simulink model "battery_model_2RC_2S1P"  (R2025a)
settings: Solver=ode15s  StartTime=0.0  StopTime=3600  RelTol=1e-2  AbsTol=1e-3  EnableMultiTasking=on
libraries: fl_lib x19, nesl_utility x17, ee_lib x4, batteryecm_lib x2
settings Model: LastModifiedBy=ishikawa
settings SolverCC: AutoScaleAbsTol=off  AlgebraicLoopSolver=TrustRegion  MaxZcPerStep=1.0
settings DataIOCC: LimitDataPoints=on  MaxDataPoints=10000
settings OptimizationCC: ReuseModelBlockBuffer=off  LifeSpan=inf
settings DebuggingCC: UnconnectedInputMsg=warning  UnconnectedOutputMsg=warning  UnconnectedLineMsg=warning  AllowSymbolicDim=off  SFUnexpectedBacktrackingDiag=warning  SFNoUnconditionalDefaultTransitionDiag=warning  SFExecutionAtInitializationDiag=none  ArithmeticOperatorsInVariantConditions=warning
settings ModelReferenceCC: EnableRefExpFcnMdlSchedulingChecks=on
settings SFSimCC: SimUseLocalCustomCode=off  CustomCodeUndefinedFunction=UseInterfaceOnly
settings RTWCC: RTWUseLocalCustomCode=off  GPUComputeCapability=3.5  DLArmComputeVersion=19.05
settings CodeAppCC: StateflowObjectComments=on
settings GRTTargetCC: TargetLangStandard=C89/C90 (ANSI)
settings ConfigComp: CovMetricSettings=dw  CovSaveCumulativeToWorkspaceVar=on  CovSaveSingleToWorkspaceVar=on  CovExternalEMLEnable=off  CovSFcnEnable=off
settings SimscapeCC: SimscapeLogType=all  SimscapeLogSimulationStatistics=on  SimscapeLogDataHistory=10000.0

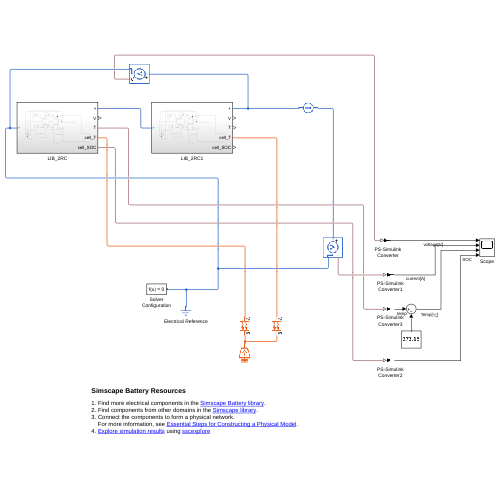
[thumbnail: Simulink's stored preview of the top-level diagram]
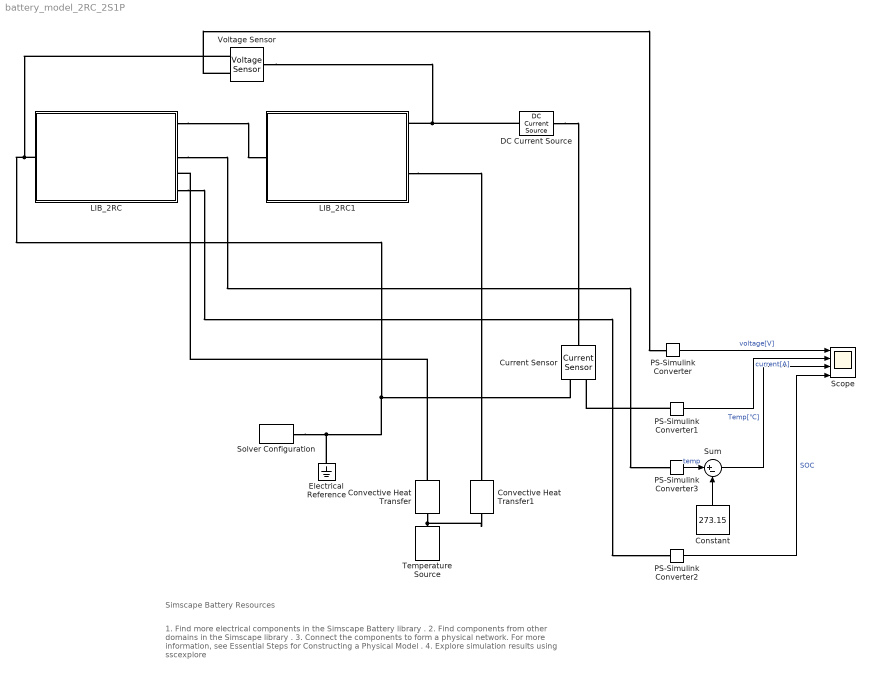
== system battery_model_2RC_2S1P ==
  note: 1. Find more electrical components in the Simscape Battery library .
      | 2. Find components from other domains in the Simscape library .
      | 3. Connect the components to form a physical network.
      | For more information, see Essential Steps for Constructing a Physical Model .
      | 4. Explore simulation results using sscexplore
  note: Simscape Battery Resources
  Constant : Constant  Value=273.15
  Convective Heat Transfer : fl_lib/Thermal/Thermal Elements/Convective Heat Transfer  thermal_type=foundation.enum.constant_variable.constant  area=4398.2 mm^2  heat_tr_coeff=20 W/(K*m^2)  min_heat_tr_coeff=1e-3 W/(K*m^2)  T_specify=off  T_priority=None  T=0 K  T_nominal_specify=off  T_nominal_value=1  T_nominal_unit=K  Q_specify=off  Q_priority=None  Q=0 W  Q_nominal_specify=off  Q_nominal_value=1  Q_nominal_unit=W
  Convective Heat Transfer1 : fl_lib/Thermal/Thermal Elements/Convective Heat Transfer  thermal_type=foundation.enum.constant_variable.constant  area=4398.2 mm^2  heat_tr_coeff=20 W/(K*m^2)  min_heat_tr_coeff=1e-3 W/(K*m^2)  T_specify=off  T_priority=None  T=0 K  T_nominal_specify=off  T_nominal_value=1  T_nominal_unit=K  Q_specify=off  Q_priority=None  Q=0 W  Q_nominal_specify=off  Q_nominal_value=1  Q_nominal_unit=W
  Current Sensor : fl_lib/Electrical/Electrical Sensors/Current Sensor
  DC Current Source : fl_lib/Electrical/Electrical Sources/DC Current Source  i0=5 A
      settings: InternalSimscapePortConfiguration="{\"Bottom\":[],\"Left\":[{\"id\":\"p\",\"label\":\"\",\"type\":\"foundation.electrical.electrical\"}],\"Right\":[{\"id\":\"n\",\"label\":\"\",\"type\":\"foundation.electrical.electrical\"}],\"Top\":[]}"
  Electrical Reference : fl_lib/Electrical/Electrical Elements/Electrical Reference
  LIB_2RC : Subsystem
  LIB_2RC1 : Subsystem
  PS-Simulink Converter{,1..3} (4 alike) : nesl_utility/PS-Simulink Converter  PhysicalDomain=network_engine_domain  SubClassName=ps_output  LeftPortType=input  RightPortType=output  PseudoPeriodic=off  Frequencies=[]  VectorFormat=inherit  Unit=inherit  AffineConversion=off
  Scope : Scope  NumInputPorts=4
      settings: ActiveDisplayYMinimum=3.6038991056085474  ActiveDisplayYMaximum=8.7134975618645871
  Solver Configuration : nesl_utility/Solver Configuration  PhysicalDomain=network_engine_domain  SubClassName=solver  LeftPortType=input  RightPortType=generic  Tones=[]  Harmonics=[]  SimulateNoise=off  Profile=off  UseLocalSampling=off  EnableSwitchedLinearOptims=on  FrequencyDomain=off  UseCCode=off  RelTol=0.001  AbsTol=1e-06  MinStep=1e-09  ToWorkspace=off  RevertToSquareIcSolve=off  NumHomotopyIterations=100  PhasorMode=off  PhasorModeNumHarmonics=1  ConsistencySolver=NEWTON_XTOL_AFTER_FTOL  IndexReductionMethod=DerivativeReplacement  DoDC=off  ResidualTolerance=1e-09  ConsistencyTolSource=GLOBAL  ConsistencyAbsTol=0.001  ConsistencyRelTol=0.001  ConsistencyTolFactor=0.001  UseLocalSolver=off  LocalSolverChoice=NE_BACKWARD_EULER_ADVANCER  ResolveIndetEquations=on  FunctionEvalNumThread=1  LocalSolverSampleTime=0.001  DoFixedCost=off  MaxNonlinIter=3  MaxModeIter=2  ComputeImpulses=off  ImpulseIterations=2  LinearAlgebra=auto  LinearAlgebraNumThread=0  EquationFormulation=NE_TIME_EF  DelaysMemoryBudget=1024  AutomaticFiltering=on  FilteringTimeConstant=0.001  PartitionStorageMethod=AS_NEEDED  PartitionMemoryBudget=1024  PartitionMethod=ROBUST  MultibodyUseLocalSolver=off  MultibodyLocalSolverChoice=ODE1  MultibodyLocalSolverSampleTime=0.001
  Sum : Sum  Inputs=|+-
  Temperature Source : fl_lib/Thermal/Thermal Sources/Temperature Source  temperature=298.15 K
  Voltage Sensor : fl_lib/Electrical/Electrical Sensors/Voltage Sensor
  wires:
  PS-Simulink Converter/1 -> Scope/1  "voltage[V]"
  PS-Simulink Converter1/1 -> Scope/2  "current[A]"
  PS-Simulink Converter2/1 -> Scope/4  "SOC"
  PS-Simulink Converter3/1 -> Sum/1  "temp"
  Constant/1 -> Sum/2
  Sum/1 -> Scope/3  "Temp[℃]"
  connections:
  Solver Configuration/RConn1 -- Electrical Reference/LConn1 -- Voltage Sensor/RConn2 -- LIB_2RC/LConn1 -- Current Sensor/RConn2
  PS-Simulink Converter1/LConn1 -- Current Sensor/RConn1
  DC Current Source/LConn1 -- Current Sensor/LConn1
  Convective Heat Transfer/RConn1 -- Convective Heat Transfer1/RConn1 -- Temperature Source/LConn1
  LIB_2RC/RConn3 -- PS-Simulink Converter3/LConn1
  Convective Heat Transfer/LConn1 -- LIB_2RC/RConn4
  LIB_2RC/RConn5 -- PS-Simulink Converter2/LConn1
  LIB_2RC/RConn1 -- LIB_2RC1/LConn1
  DC Current Source/RConn1 -- Voltage Sensor/LConn1 -- LIB_2RC1/RConn1
  Voltage Sensor/RConn1 -- PS-Simulink Converter/LConn1
  LIB_2RC1/RConn4 -- Convective Heat Transfer1/LConn1

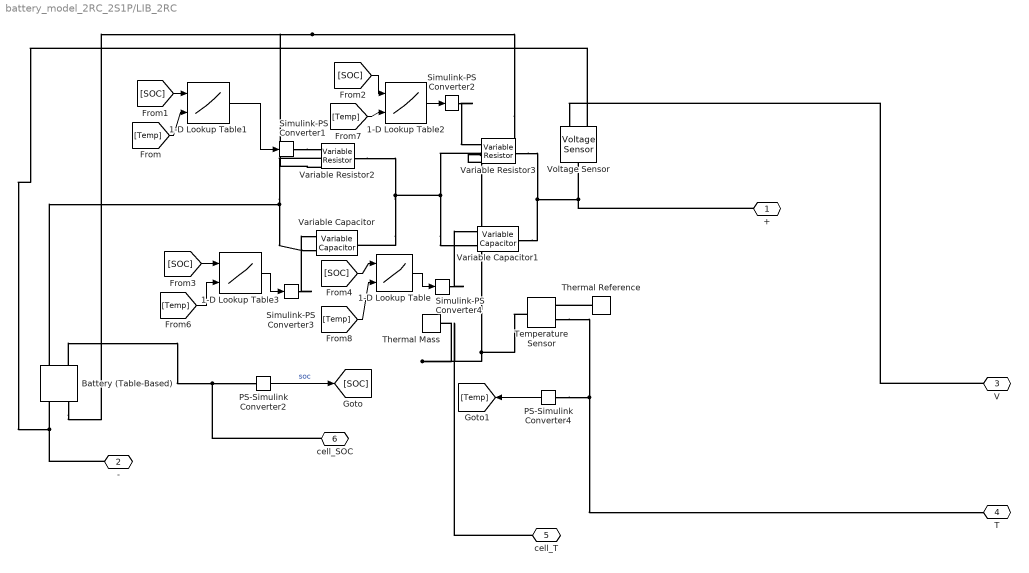
== system battery_model_2RC_2S1P/LIB_2RC ==
  1-D Lookup Table : Lookup_n-D  BreakpointsForDimension1=[0.2;0.3;0.4;0.5;0.6;0.7;0.8]  BreakpointsForDimension2=[243.15;253.15;263.15;273.15;293.15;313.15;333.15]  Table=[397.027539766071 413.310716720776 450.288774751873 484.819114610467 708.496704080481 1018.18115313393 1458.65326678376;424.160278757141 453.825413446659 523.404522348996 631.9600040269009 947.03250742128 1493.43845540211 2217.48074264787;445.080170656404 486.033224095827 563.317756801399 683.004425228606 1038.61139579099 1674.11304631932 2558.22434329923;455.398203100465 496.827822276761 571.533663638549 690.280792821343 1055.52640859521 1694.30417810877 2606.65823475404;450.805024482046 491.645093905588 567.6042393287059 687.869379202455 958.88347532501 1503.12492310199 2245.84613474158;459.20425063845 505.517182572026 566.7462150739819 674.399780009527 1012.81365894071 1541.62099228793 2186.17014175407;440.690556106675 465.368272327513 510.221909646828 603.247409685859 936.9228291323921 1585.76440619997 2335.62274337301]  InterpMethod=Cubic spline  ExtrapMethod=Cubic spline  InternalRulePriority=Speed  RndMeth=Simplest
      settings: InputPortMap=u0,u1
  1-D Lookup Table1 : Lookup_n-D  BreakpointsForDimension1=[0.1;0.2;0.3;0.4;0.5;0.6;0.7;0.8;0.9]  BreakpointsForDimension2=[243.15;253.15;263.15;273.15;293.15;313.15;333.15]  Table=[0.0648840256616996 0.0548544229488452 0.0410756789651543 0.00365935665197351 0.00410447217653615 0.0042287075329693 0.00446198100466879;0.000100000000000031 0.000185860329266272 0.00063291627023489 0.000604389587689878 0.00159168669392803 0.0016313368228375 0.00200106459466915;0.000100000000000657 0.000178858598639097 0.000694707150185237 0.00125188824704277 0.00176891372610466 0.00209070161735659 0.00247958451818985;0.000100000000001458 0.000100000085659489 0.000423782841219483 0.000938984921591674 0.00141231326940913 0.00167345242239196 0.00202829350359598;0.000100000000005779 0.000100000434574669 0.000364143335480069 0.0009126326610232501 0.00147302896089186 0.00170156587463233 0.0020630219200505;0.000100000000000059 0.000278496083040111 0.000932087348991903 0.00158899396065768 0.00191094085461356 0.00241949669919031 0.00294718757231742;0.000157820659890285 0.00106750348889988 0.00170837536179057 0.00230532371700022 0.00287920920827158 0.00321022629451256 0.00313048840253092;0.00177370275978769 0.00220599934990951 0.00213979379110787 0.00196046296256981 0.00192605061749151 0.00211861368543494 0.00233113190320715;0.000100000002763379 0.000100000000000054 0.000100000000653121 0.0001 0.008148072217938821 0.000704666332425065 0.00115546872752894]  InternalRulePriority=Speed  RndMeth=Simplest
      settings: InputPortMap=u0,u1
  1-D Lookup Table2 : Lookup_n-D  BreakpointsForDimension1=[0.1;0.2;0.3;0.4;0.5;0.6;0.7;0.8;0.9]  BreakpointsForDimension2=[243.15;253.15;263.15;273.15;293.15;313.15;333.15]  Table=[0.0312362200904875 0.0315941026250706 0.0325412525306707 0.06566459208756791 0.0513687856330062 0.0398557955825684 0.0352414860805867;0.0583154306341024 0.0541889718032672 0.0485485115411798 0.0405853877005846 0.0253230417200522 0.0179009478462281 0.014307904930947;0.0536064189215573 0.0500390783463631 0.0433999709749259 0.0362267299181839 0.0236360991500641 0.0163691636487888 0.0130777917670481;0.0510050016137325 0.0473244390449334 0.0406214407925902 0.0337999790008502 0.0217500314411443 0.014239465970092 0.0108482476470579;0.0489305258721882 0.0456158921911874 0.0395186949619077 0.032565240420024 0.0203018907734851 0.0132138263566234 0.0100754346546588;0.052109451999107 0.049581529928274 0.0435904805430911 0.0359457745514755 0.0223175296306251 0.0168395096404479 0.0145466336811264;0.0464891543332739 0.0461866422714133 0.0413831033248225 0.0343229536328831 0.0214923117112032 0.0152124572665625 0.012597749276845;0.0507650491686061 0.0490964567145729 0.0447555398141767 0.0371516971280947 0.0236401140020694 0.0168783192334412 0.0134119198713262;0.0485073831147304 0.0352842403123327 0.0287671376669305 0.0265741690411721 0.0113474189770295 0.0120077119241438 0.00910795807643172]  InternalRulePriority=Speed  RndMeth=Simplest
      settings: InputPortMap=u0,u1
  1-D Lookup Table3 : Lookup_n-D  BreakpointsForDimension1=[0.1;0.2;0.3;0.4;0.5;0.6;0.7;0.8;0.9]  BreakpointsForDimension2=[243.15;253.15;263.15;273.15;293.15;313.15;333.15]  Table=[424.737364805381 483.271376452374 636.374167822421 110.165370185585 210.959116483621 313.2910014267 429.704220236589;52.6100971695542 105.248860126284 63.6650097826792 60.5918177276404 590.998027541052 996.160700447975 1154.49089964508;90.42580825145249 312.74974100652 48.6954548231183 44.3380567111186 357.175111931739 582.326548341105 771.438129167261;118.248383199082 99.28484606029799 166.076514539697 33.3725870856565 424.226062352995 719.387999873913 951.14636655943;918.679938144521 17.7650082120618 162.910459604258 69.3161002074154 489.546217553075 740.276114872735 939.308771982209;2.33207460618265 21.5530951458301 3.6964219785336 146.524187256498 348.153708802123 510.139939288567 656.967471434281;531.457927571111 27.4074025424315 2.72381788457468 199.034282888046 301.850047314288 496.97606871071 792.228617026462;17.756055458357 149.39468287018 289.425440553852 448.824396398649 673.5667264432579 937.09993120302 1096.43767182893;134.492899453975 350.115225919153 316.422261704154 264.245690439253 3346.03757120953 1441.63234506984 1579.79386522281]  InternalRulePriority=Speed  RndMeth=Simplest
      settings: InputPortMap=u0,u1
  Battery (Table-Based) : batteryecm_lib/Battery (Table-Based)  SOC_vec=[0, .2, .4, .6, .8, 1 ]  T_dependence=simscape.enum.tablebattery.temperature_dependence.yes  prm_dir=simscape.enum.tablebattery.prm_dir.noCurrentDirectionality  T_vec=[243.15, 273.15, 333.15] K  V0_mat="[2.5, 2.5, 2.5; 3.42101188834904, 3.429363958294, 3.43097550824307; 3.59742438009383, 3.61108748742895, 3.6176423842731; 3.78966665741075, 3.80246978402262, 3.81751594086923;  4.00549793710987, 4.02037931005492, 4.02637725260671; 4.2, 4.2, 4.2] V"  V0_vec=[3.5057, 3.566, 3.6337, 3.7127, 3.9259, 4.0777, 4.1928] V  V_range=[0, inf] V  R0_mat=[0.14, 0.053, 0.008; 0.129999964197049, 0.0446688648295249, 0.00668298362381311; 0.116587668750708, 0.0373578823461791, 0.00550858692009345; 0.108099281225994, 0.0323106583204613, 0.00506405532754667; 0.104972042746652, 0.0314197816681482, 0.00495762078874784; 0.105, 0.031, 0.00495 ] Ohm  R0_vec=[.0085, .0085, .0087, .0082, .0083, .0085, .0085] Ohm  R0_dis_mat=[.0117, .0085, .009; .011, .0085, .009; .0114, .0087, .0092; .0107, .0082, .0088; .0107, .0083, .0091; .0113, .0085, .0089; .0116, .0085, .0089] Ohm  R0_dis_vec=[.0085, .0085, .0087, .0082, .0083, .0085, .0085] Ohm  R0_ch_mat=[.0117, .0085, .009; .011, .0085, .009; .0114, .0087, .0092; .0107, .0082, .0088; .0107, .0083, .0091; .0113, .0085, .0089; .0116, .0085, .0089] Ohm  R0_ch_vec=[.0085, .0085, .0087, .0082, .0083, .0085, .0085] Ohm  AH=5 A*hr  prm_leak=simscape.enum.tablebattery.prm_leak.disabled  Rleak_vec=[8000, 7000, 6000] Ohm  Rleak=7e3 Ohm  extrapolation_option=simscape.enum.extrapolation.nearest  SOC_port=simscape.enum.tablebattery.enable.yes  prm_dyn=simscape.enum.tablebattery.prm_dyn.off  R1_mat=[.0109, .0029, .0013; .0069, .0024, .0012; .0047, .0026, .0013; .0034, .0016, .001; .0033, .0023, .0014; .0033, .0018, .0011; .0028, .0017, .0011] Ohm  R1_vec=[.0029, .0024, .0026, .0016, .0023, .0018, .0017] Ohm  tau1_mat=[20, 36, 39; 31, 45, 39; 109, 105, 61; 36, 29, 26; 59, 77, 67; 40, 33, 29; 25, 39, 33] s  tau1_vec=[36, 45, 105, 29, 77, 33, 39] s  R2_mat=[.0109, .0029, .0013; .0069, .0024, .0012; .0047, .0026, .0013; .0034, .0016, .001; .0033, .0023, .0014; .0033, .0018, .0011; .0028, .0017, .0011] Ohm  R2_vec=[.0029, .0024, .0026, .0016, .0023, .0018, .0017] Ohm  tau2_mat=[20, 36, 39; 31, 45, 39; 109, 105, 61; 36, 29, 26; 59, 77, 67; 40, 33, 29; 25, 39, 33] s  tau2_vec=[36, 45, 105, 29, 77, 33, 39] s  R3_mat=[.0109, .0029, .0013; .0069, .0024, .0012; .0047, .0026, .0013; .0034, .0016, .001; .0033, .0023, .0014; .0033, .0018, .0011; .0028, .0017, .0011] Ohm  R3_vec=[.0029, .0024, .0026, .0016, .0023, .0018, .0017] Ohm  tau3_mat=[20, 36, 39; 31, 45, 39; 109, 105, 61; 36, 29, 26; 59, 77, 67; 40, 33, 29; 25, 39, 33] s  tau3_vec=[36, 45, 105, 29, 77, 33, 39] s  R4_mat=[.0109, .0029, .0013; .0069, .0024, .0012; .0047, .0026, .0013; .0034, .0016, .001; .0033, .0023, .0014; .0033, .0018, .0011; .0028, .0017, .0011] Ohm  R4_vec=[.0029, .0024, .0026, .0016, .0023, .0018, .0017] Ohm  tau4_mat=[20, 36, 39; 31, 45, 39; 109, 105, 61; 36, 29, 26; 59, 77, 67; 40, 33, 29; 25, 39, 33] s  tau4_vec=[36, 45, 105, 29, 77, 33, 39] s  R5_mat=[.0109, .0029, .0013; .0069, .0024, .0012; .0047, .0026, .0013; .0034, .0016, .001; .0033, .0023, .0014; .0033, .0018, .0011; .0028, .0017, .0011] Ohm  R5_vec=[.0029, .0024, .0026, .0016, .0023, .0018, .0017] Ohm  tau5_mat=[20, 36, 39; 31, 45, 39; 109, 105, 61; 36, 29, 26; 59, 77, 67; 40, 33, 29; 25, 39, 33] s  tau5_vec=[36, 45, 105, 29, 77, 33, 39] s  prm_fade=simscape.enum.tablebattery.prm_fade.equations  N0=100  dV0=0  dR0=0  dAH=0  dRleak=0  dR1=0  dR2=0  dR3=0  dR4=0  dR5=0  N0vec=[100, 200, 300]  Tfadevec=[298.15, 323.15] K  dV0vec=[0, 0, 0]  dR0vec=[0, 0, 0]  dAHvec=[0, 0, 0]  dRleakvec=[0, 0, 0]  dR1vec=[0, 0, 0]  dR2vec=[0, 0, 0]  dR3vec=[0, 0, 0]  dR4vec=[0, 0, 0]  dR5vec=[0, 0, 0]  dV0mat=[0, 0; 0, 0; 0, 0]  dR0mat=[0, 0; 0, 0; 0, 0]  dAHmat=[0, 0; 0, 0; 0, 0]  dRleakmat=[0, 0; 0, 0; 0, 0]  dR1mat=[0, 0; 0, 0; 0, 0]  dR2mat=[0, 0; 0, 0; 0, 0]  dR3mat=[0, 0; 0, 0; 0, 0]  dR4mat=[0, 0; 0, 0; 0, 0]  dR5mat=[0, 0; 0, 0; 0, 0]  prm_age_modeling=simscape.enum.tablebattery.prm_age_modeling.equation  storage_dt_age_vec=[0] d  storage_T_age_vec=[273] K  prm_age_OCV=simscape.enum.tablebattery.prm_age_OCV.OCV  OCV_age=0.9  SOC_age=0.6  prm_age_resistance=simscape.enum.tablebattery.prm_age.disabled  OCV_scaling_age_resistance=2.2134e6  OCV_offset_age_resistance=1.632e6  temp_exp_age_resistance=0.515833569 V  t_exp_age_resistance=0.75  T_age_vec_resistance=[273.15, 298.15, 323.15] K  dt_age_vec_resistance=[90, 180, 270, 360] d  dR0_age_vec=[0, 0, 0]  t_meas_dR0_age=100 d  dR0_age_mat=[0, 0, 0; 0, 0, 0; 0, 0, 0; 0, 0, 0]  prm_age_capacity=simscape.enum.tablebattery.prm_age.disabled  OCV_scaling_age_capacity=1.5097e07  OCV_offset_age_capacity=8.3625e06  temp_exp_age_capacity=0.6011 V  t_exp_age_capacity=0.75  T_age_vec_capacity=[273.15, 298.15, 323.15] K  dt_age_vec_capacity=[90, 180, 270, 360] d  dAH_age_vec=[0, 0, 0]  t_meas_dAH_age=100 d  dAH_age_mat=[0, 0, 0; 0, 0, 0; 0, 0, 0; 0, 0, 0]  thermal_port=simscape.enum.thermaleffects.model  temperature=298.15 K  thermal_mass=1 J/K  i_specify=off  i_priority=None  i=0 A  i_nominal_specify=off  i_nominal_value=1  i_nominal_unit=A  v_specify=off  v_priority=None  v=0 V  v_nominal_specify=off  v_nominal_value=1  v_nominal_unit=V  stateOfCharge_specify=on  stateOfCharge_priority=High  stateOfCharge=1  stateOfCharge_nominal_specify=on  stateOfCharge_nominal_value=1  stateOfCharge_nominal_unit=1  num_cycles_specify=off  num_cycles_priority=High  num_cycles=0  num_cycles_nominal_specify=off  num_cycles_nominal_value=1  num_cycles_nominal_unit=1  cell_temperature_specify=on  cell_temperature_priority=High  cell_temperature=298.15 K  cell_temperature_nominal_specify=off  cell_temperature_nominal_value=1  cell_temperature_nominal_unit=K
  PS-Simulink Converter2 : nesl_utility/PS-Simulink Converter  PhysicalDomain=network_engine_domain  SubClassName=ps_output  LeftPortType=input  RightPortType=output  PseudoPeriodic=off  Frequencies=[]  VectorFormat=inherit  Unit=inherit  AffineConversion=off
  PS-Simulink Converter4 : nesl_utility/PS-Simulink Converter  PhysicalDomain=network_engine_domain  SubClassName=ps_output  LeftPortType=input  RightPortType=output  PseudoPeriodic=off  Frequencies=[]  VectorFormat=inherit  Unit=inherit  AffineConversion=off
  Simulink-PS Converter{1..4} (4 alike) : nesl_utility/Simulink-PS Converter  PhysicalDomain=network_engine_domain  SubClassName=ps_input  LeftPortType=input  RightPortType=output  PseudoPeriodic=off  Frequencies=[]  NoiseDistribution=none  NoiseParameters=[]  Unit=1  AffineConversion=off  FilteringAndDerivatives=provide  SimscapeFilterOrder=1  InputFilterTimeConstant=0.001  UdotUserProvided=0
  Temperature Sensor : fl_lib/Thermal/Thermal Sensors/Temperature Sensor  temperature_measure=foundation.enum.MeasurementReference.difference
  Thermal Mass : fl_lib/Thermal/Thermal Elements/Thermal Mass  mass_type=foundation.enum.constant_variable.constant  mass=67.9 g  sp_heat=900 J/(K*kg)  mass_min=1e-6 kg  num_ports=foundation.enum.numPorts2.one  m_specify=off  m_priority=High  m=1 kg  m_nominal_specify=off  m_nominal_value=1  m_nominal_unit=kg  T_specify=off  T_priority=High  T=300 K  T_nominal_specify=off  T_nominal_value=1  T_nominal_unit=K  Q_specify=off  Q_priority=None  Q=0 W  Q_nominal_specify=off  Q_nominal_value=1  Q_nominal_unit=W
  Thermal Reference : fl_lib/Thermal/Thermal Elements/Thermal Reference
  Variable Capacitor : ee_lib/Passive/Variable Capacitor  prm=2  Cmin=1e-9 F  r=1e-6 Ohm  v0=0 V  q0=0 C
      settings: InternalSimscapePortConfiguration="{\"Bottom\":[],\"Left\":[{\"id\":\"C\",\"label\":\"C\",\"type\":\"input\"},{\"id\":\"p\",\"label\":\"+\",\"type\":\"foundation.electrical.electrical\"}],\"Right\":[{\"id\":\"n\",\"label\":\"-\",\"type\":\"foundation.electrical.electrical\"}],\"Top\":[]}"
  Variable Capacitor1 : ee_lib/Passive/Variable Capacitor  prm=2  Cmin=1e-9 F  r=1e-6 Ohm  v0=0 V  q0=0 C
      settings: InternalSimscapePortConfiguration="{\"Bottom\":[],\"Left\":[{\"id\":\"C\",\"label\":\"C\",\"type\":\"input\"},{\"id\":\"p\",\"label\":\"+\",\"type\":\"foundation.electrical.electrical\"}],\"Right\":[{\"id\":\"n\",\"label\":\"-\",\"type\":\"foundation.electrical.electrical\"}],\"Top\":[]}"
  Variable Resistor2 : fl_lib/Electrical/Electrical Elements/Variable Resistor  Rmin=0 Ohm  thermalEnable=true  thermal_mass=1 J/K  i_specify=off  i_priority=None  i=0 A  i_nominal_specify=off  i_nominal_value=1  i_nominal_unit=A  v_specify=off  v_priority=None  v=0 V  v_nominal_specify=off  v_nominal_value=1  v_nominal_unit=V  T_specify=off  T_priority=None  T=300 K  T_nominal_specify=off  T_nominal_value=1  T_nominal_unit=K
      settings: InternalSimscapePortConfiguration="{\"Bottom\":[],\"Left\":[{\"id\":\"R\",\"label\":\"R\",\"type\":\"input\"},{\"id\":\"p\",\"label\":\"+\",\"type\":\"foundation.electrical.electrical\"}],\"Right\":[{\"id\":\"n\",\"label\":\"-\",\"type\":\"foundation.electrical.electrical\"}],\"Top\":[{\"id\":\"H\",\"label\":\"H\",\"type\":\"foundation.thermal.thermal\"}]}"
  Variable Resistor3 : fl_lib/Electrical/Electrical Elements/Variable Resistor  Rmin=0 Ohm  thermalEnable=true  thermal_mass=1 J/K  i_specify=off  i_priority=None  i=0 A  i_nominal_specify=off  i_nominal_value=1  i_nominal_unit=A  v_specify=off  v_priority=None  v=0 V  v_nominal_specify=off  v_nominal_value=1  v_nominal_unit=V  T_specify=off  T_priority=None  T=300 K  T_nominal_specify=off  T_nominal_value=1  T_nominal_unit=K
      settings: InternalSimscapePortConfiguration="{\"Bottom\":[],\"Left\":[{\"id\":\"R\",\"label\":\"R\",\"type\":\"input\"},{\"id\":\"p\",\"label\":\"+\",\"type\":\"foundation.electrical.electrical\"}],\"Right\":[{\"id\":\"n\",\"label\":\"-\",\"type\":\"foundation.electrical.electrical\"}],\"Top\":[{\"id\":\"H\",\"label\":\"H\",\"type\":\"foundation.thermal.thermal\"}]}"
  Voltage Sensor : fl_lib/Electrical/Electrical Sensors/Voltage Sensor
  + : PMIOPort  Side=Right
  - : PMIOPort  Port=2  Side=Left
  V : PMIOPort  Port=3  Side=Right
  T : PMIOPort  Port=4  Side=Right
  cell_T : PMIOPort  Port=5  Side=Right
  cell_SOC : PMIOPort  Port=6  Side=Right
  wires:
  [SOC] -> 1-D Lookup Table/1
  1-D Lookup Table1/1 -> Simulink-PS Converter1/1
  PS-Simulink Converter4/1 -> [Temp]
  [Temp] -> 1-D Lookup Table3/2
  [SOC] -> 1-D Lookup Table2/1
  [SOC] -> 1-D Lookup Table1/1
  1-D Lookup Table3/1 -> Simulink-PS Converter3/1
  [SOC] -> 1-D Lookup Table3/1
  [Temp] -> 1-D Lookup Table1/2
  [Temp] -> 1-D Lookup Table2/2
  [Temp] -> 1-D Lookup Table/2
  PS-Simulink Converter2/1 -> [SOC]  "soc"
  1-D Lookup Table2/1 -> Simulink-PS Converter2/1
  1-D Lookup Table/1 -> Simulink-PS Converter4/1
  connections:
  Battery (Table-Based)/LConn2 -- cell_SOC/RConn1 -- PS-Simulink Converter2/LConn1
  Variable Capacitor/LConn2 -- Battery (Table-Based)/LConn1 -- Variable Resistor2/LConn2
  Temperature Sensor/RConn2 -- T/RConn1 -- PS-Simulink Converter4/LConn1
  -/RConn1 -- Voltage Sensor/RConn2 -- Battery (Table-Based)/RConn1
  V/RConn1 -- Voltage Sensor/RConn1
  Simulink-PS Converter3/RConn1 -- Variable Capacitor/LConn1
  Simulink-PS Converter4/RConn1 -- Variable Capacitor1/LConn1
  Thermal Reference/LConn1 -- Temperature Sensor/RConn1
  Variable Resistor3/LConn2 -- Variable Capacitor/RConn1 -- Variable Resistor2/RConn1 -- Variable Capacitor1/LConn2
  Simulink-PS Converter1/RConn1 -- Variable Resistor2/LConn1
  Simulink-PS Converter2/RConn1 -- Variable Resistor3/LConn1
  Variable Capacitor1/RConn1 -- Variable Resistor3/RConn1 -- +/RConn1 -- Voltage Sensor/LConn1
  Variable Resistor3/LConn3 -- Variable Resistor2/LConn3 -- Battery (Table-Based)/RConn2 -- Temperature Sensor/LConn1 -- cell_T/RConn1 -- Thermal Mass/LConn1

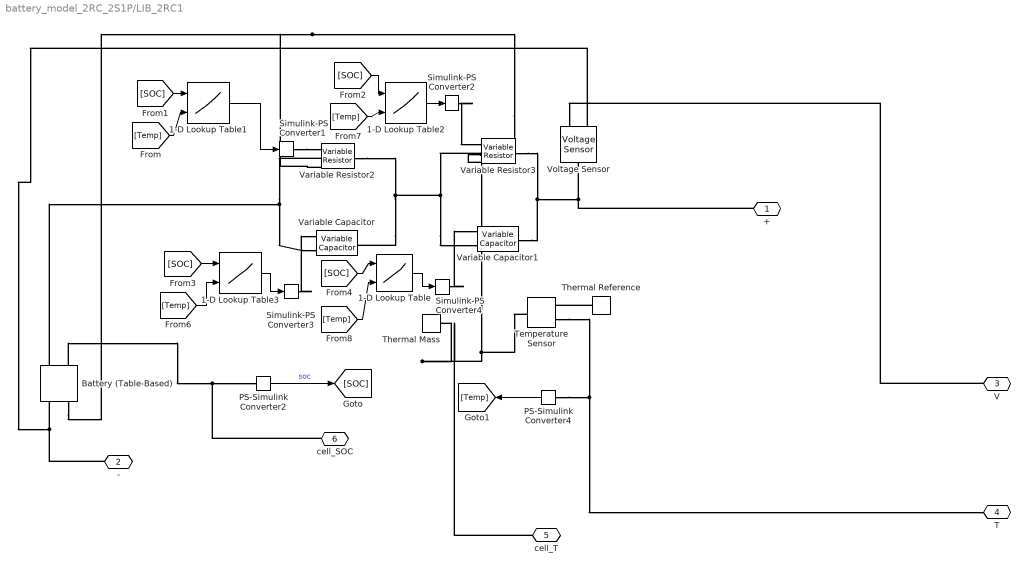
== system battery_model_2RC_2S1P/LIB_2RC1 ==
  1-D Lookup Table : Lookup_n-D  BreakpointsForDimension1=[0.2;0.3;0.4;0.5;0.6;0.7;0.8]  BreakpointsForDimension2=[243.15;253.15;263.15;273.15;293.15;313.15;333.15]  Table=[397.027539766071 413.310716720776 450.288774751873 484.819114610467 708.496704080481 1018.18115313393 1458.65326678376;424.160278757141 453.825413446659 523.404522348996 631.9600040269009 947.03250742128 1493.43845540211 2217.48074264787;445.080170656404 486.033224095827 563.317756801399 683.004425228606 1038.61139579099 1674.11304631932 2558.22434329923;455.398203100465 496.827822276761 571.533663638549 690.280792821343 1055.52640859521 1694.30417810877 2606.65823475404;450.805024482046 491.645093905588 567.6042393287059 687.869379202455 958.88347532501 1503.12492310199 2245.84613474158;459.20425063845 505.517182572026 566.7462150739819 674.399780009527 1012.81365894071 1541.62099228793 2186.17014175407;440.690556106675 465.368272327513 510.221909646828 603.247409685859 936.9228291323921 1585.76440619997 2335.62274337301]  InterpMethod=Cubic spline  ExtrapMethod=Cubic spline  InternalRulePriority=Speed  RndMeth=Simplest
      settings: InputPortMap=u0,u1
  1-D Lookup Table1 : Lookup_n-D  BreakpointsForDimension1=[0.1;0.2;0.3;0.4;0.5;0.6;0.7;0.8;0.9]  BreakpointsForDimension2=[243.15;253.15;263.15;273.15;293.15;313.15;333.15]  Table=[0.0648840256616996 0.0548544229488452 0.0410756789651543 0.00365935665197351 0.00410447217653615 0.0042287075329693 0.00446198100466879;0.000100000000000031 0.000185860329266272 0.00063291627023489 0.000604389587689878 0.00159168669392803 0.0016313368228375 0.00200106459466915;0.000100000000000657 0.000178858598639097 0.000694707150185237 0.00125188824704277 0.00176891372610466 0.00209070161735659 0.00247958451818985;0.000100000000001458 0.000100000085659489 0.000423782841219483 0.000938984921591674 0.00141231326940913 0.00167345242239196 0.00202829350359598;0.000100000000005779 0.000100000434574669 0.000364143335480069 0.0009126326610232501 0.00147302896089186 0.00170156587463233 0.0020630219200505;0.000100000000000059 0.000278496083040111 0.000932087348991903 0.00158899396065768 0.00191094085461356 0.00241949669919031 0.00294718757231742;0.000157820659890285 0.00106750348889988 0.00170837536179057 0.00230532371700022 0.00287920920827158 0.00321022629451256 0.00313048840253092;0.00177370275978769 0.00220599934990951 0.00213979379110787 0.00196046296256981 0.00192605061749151 0.00211861368543494 0.00233113190320715;0.000100000002763379 0.000100000000000054 0.000100000000653121 0.0001 0.008148072217938821 0.000704666332425065 0.00115546872752894]  InternalRulePriority=Speed  RndMeth=Simplest
      settings: InputPortMap=u0,u1
  1-D Lookup Table2 : Lookup_n-D  BreakpointsForDimension1=[0.1;0.2;0.3;0.4;0.5;0.6;0.7;0.8;0.9]  BreakpointsForDimension2=[243.15;253.15;263.15;273.15;293.15;313.15;333.15]  Table=[0.0312362200904875 0.0315941026250706 0.0325412525306707 0.06566459208756791 0.0513687856330062 0.0398557955825684 0.0352414860805867;0.0583154306341024 0.0541889718032672 0.0485485115411798 0.0405853877005846 0.0253230417200522 0.0179009478462281 0.014307904930947;0.0536064189215573 0.0500390783463631 0.0433999709749259 0.0362267299181839 0.0236360991500641 0.0163691636487888 0.0130777917670481;0.0510050016137325 0.0473244390449334 0.0406214407925902 0.0337999790008502 0.0217500314411443 0.014239465970092 0.0108482476470579;0.0489305258721882 0.0456158921911874 0.0395186949619077 0.032565240420024 0.0203018907734851 0.0132138263566234 0.0100754346546588;0.052109451999107 0.049581529928274 0.0435904805430911 0.0359457745514755 0.0223175296306251 0.0168395096404479 0.0145466336811264;0.0464891543332739 0.0461866422714133 0.0413831033248225 0.0343229536328831 0.0214923117112032 0.0152124572665625 0.012597749276845;0.0507650491686061 0.0490964567145729 0.0447555398141767 0.0371516971280947 0.0236401140020694 0.0168783192334412 0.0134119198713262;0.0485073831147304 0.0352842403123327 0.0287671376669305 0.0265741690411721 0.0113474189770295 0.0120077119241438 0.00910795807643172]  InternalRulePriority=Speed  RndMeth=Simplest
      settings: InputPortMap=u0,u1
  1-D Lookup Table3 : Lookup_n-D  BreakpointsForDimension1=[0.1;0.2;0.3;0.4;0.5;0.6;0.7;0.8;0.9]  BreakpointsForDimension2=[243.15;253.15;263.15;273.15;293.15;313.15;333.15]  Table=[424.737364805381 483.271376452374 636.374167822421 110.165370185585 210.959116483621 313.2910014267 429.704220236589;52.6100971695542 105.248860126284 63.6650097826792 60.5918177276404 590.998027541052 996.160700447975 1154.49089964508;90.42580825145249 312.74974100652 48.6954548231183 44.3380567111186 357.175111931739 582.326548341105 771.438129167261;118.248383199082 99.28484606029799 166.076514539697 33.3725870856565 424.226062352995 719.387999873913 951.14636655943;918.679938144521 17.7650082120618 162.910459604258 69.3161002074154 489.546217553075 740.276114872735 939.308771982209;2.33207460618265 21.5530951458301 3.6964219785336 146.524187256498 348.153708802123 510.139939288567 656.967471434281;531.457927571111 27.4074025424315 2.72381788457468 199.034282888046 301.850047314288 496.97606871071 792.228617026462;17.756055458357 149.39468287018 289.425440553852 448.824396398649 673.5667264432579 937.09993120302 1096.43767182893;134.492899453975 350.115225919153 316.422261704154 264.245690439253 3346.03757120953 1441.63234506984 1579.79386522281]  InternalRulePriority=Speed  RndMeth=Simplest
      settings: InputPortMap=u0,u1
  Battery (Table-Based) : batteryecm_lib/Battery (Table-Based)  SOC_vec=[0, .2, .4, .6, .8, 1 ]  T_dependence=simscape.enum.tablebattery.temperature_dependence.yes  prm_dir=simscape.enum.tablebattery.prm_dir.noCurrentDirectionality  T_vec=[243.15, 273.15, 333.15] K  V0_mat="[2.5, 2.5, 2.5; 3.42101188834904, 3.429363958294, 3.43097550824307; 3.59742438009383, 3.61108748742895, 3.6176423842731; 3.78966665741075, 3.80246978402262, 3.81751594086923;  4.00549793710987, 4.02037931005492, 4.02637725260671; 4.2, 4.2, 4.2] V"  V0_vec=[3.5057, 3.566, 3.6337, 3.7127, 3.9259, 4.0777, 4.1928] V  V_range=[0, inf] V  R0_mat=[0.14, 0.053, 0.008; 0.129999964197049, 0.0446688648295249, 0.00668298362381311; 0.116587668750708, 0.0373578823461791, 0.00550858692009345; 0.108099281225994, 0.0323106583204613, 0.00506405532754667; 0.104972042746652, 0.0314197816681482, 0.00495762078874784; 0.105, 0.031, 0.00495 ] Ohm  R0_vec=[.0085, .0085, .0087, .0082, .0083, .0085, .0085] Ohm  R0_dis_mat=[.0117, .0085, .009; .011, .0085, .009; .0114, .0087, .0092; .0107, .0082, .0088; .0107, .0083, .0091; .0113, .0085, .0089; .0116, .0085, .0089] Ohm  R0_dis_vec=[.0085, .0085, .0087, .0082, .0083, .0085, .0085] Ohm  R0_ch_mat=[.0117, .0085, .009; .011, .0085, .009; .0114, .0087, .0092; .0107, .0082, .0088; .0107, .0083, .0091; .0113, .0085, .0089; .0116, .0085, .0089] Ohm  R0_ch_vec=[.0085, .0085, .0087, .0082, .0083, .0085, .0085] Ohm  AH=5 A*hr  prm_leak=simscape.enum.tablebattery.prm_leak.disabled  Rleak_vec=[8000, 7000, 6000] Ohm  Rleak=7e3 Ohm  extrapolation_option=simscape.enum.extrapolation.nearest  SOC_port=simscape.enum.tablebattery.enable.yes  prm_dyn=simscape.enum.tablebattery.prm_dyn.off  R1_mat=[.0109, .0029, .0013; .0069, .0024, .0012; .0047, .0026, .0013; .0034, .0016, .001; .0033, .0023, .0014; .0033, .0018, .0011; .0028, .0017, .0011] Ohm  R1_vec=[.0029, .0024, .0026, .0016, .0023, .0018, .0017] Ohm  tau1_mat=[20, 36, 39; 31, 45, 39; 109, 105, 61; 36, 29, 26; 59, 77, 67; 40, 33, 29; 25, 39, 33] s  tau1_vec=[36, 45, 105, 29, 77, 33, 39] s  R2_mat=[.0109, .0029, .0013; .0069, .0024, .0012; .0047, .0026, .0013; .0034, .0016, .001; .0033, .0023, .0014; .0033, .0018, .0011; .0028, .0017, .0011] Ohm  R2_vec=[.0029, .0024, .0026, .0016, .0023, .0018, .0017] Ohm  tau2_mat=[20, 36, 39; 31, 45, 39; 109, 105, 61; 36, 29, 26; 59, 77, 67; 40, 33, 29; 25, 39, 33] s  tau2_vec=[36, 45, 105, 29, 77, 33, 39] s  R3_mat=[.0109, .0029, .0013; .0069, .0024, .0012; .0047, .0026, .0013; .0034, .0016, .001; .0033, .0023, .0014; .0033, .0018, .0011; .0028, .0017, .0011] Ohm  R3_vec=[.0029, .0024, .0026, .0016, .0023, .0018, .0017] Ohm  tau3_mat=[20, 36, 39; 31, 45, 39; 109, 105, 61; 36, 29, 26; 59, 77, 67; 40, 33, 29; 25, 39, 33] s  tau3_vec=[36, 45, 105, 29, 77, 33, 39] s  R4_mat=[.0109, .0029, .0013; .0069, .0024, .0012; .0047, .0026, .0013; .0034, .0016, .001; .0033, .0023, .0014; .0033, .0018, .0011; .0028, .0017, .0011] Ohm  R4_vec=[.0029, .0024, .0026, .0016, .0023, .0018, .0017] Ohm  tau4_mat=[20, 36, 39; 31, 45, 39; 109, 105, 61; 36, 29, 26; 59, 77, 67; 40, 33, 29; 25, 39, 33] s  tau4_vec=[36, 45, 105, 29, 77, 33, 39] s  R5_mat=[.0109, .0029, .0013; .0069, .0024, .0012; .0047, .0026, .0013; .0034, .0016, .001; .0033, .0023, .0014; .0033, .0018, .0011; .0028, .0017, .0011] Ohm  R5_vec=[.0029, .0024, .0026, .0016, .0023, .0018, .0017] Ohm  tau5_mat=[20, 36, 39; 31, 45, 39; 109, 105, 61; 36, 29, 26; 59, 77, 67; 40, 33, 29; 25, 39, 33] s  tau5_vec=[36, 45, 105, 29, 77, 33, 39] s  prm_fade=simscape.enum.tablebattery.prm_fade.equations  N0=100  dV0=0  dR0=0  dAH=0  dRleak=0  dR1=0  dR2=0  dR3=0  dR4=0  dR5=0  N0vec=[100, 200, 300]  Tfadevec=[298.15, 323.15] K  dV0vec=[0, 0, 0]  dR0vec=[0, 0, 0]  dAHvec=[0, 0, 0]  dRleakvec=[0, 0, 0]  dR1vec=[0, 0, 0]  dR2vec=[0, 0, 0]  dR3vec=[0, 0, 0]  dR4vec=[0, 0, 0]  dR5vec=[0, 0, 0]  dV0mat=[0, 0; 0, 0; 0, 0]  dR0mat=[0, 0; 0, 0; 0, 0]  dAHmat=[0, 0; 0, 0; 0, 0]  dRleakmat=[0, 0; 0, 0; 0, 0]  dR1mat=[0, 0; 0, 0; 0, 0]  dR2mat=[0, 0; 0, 0; 0, 0]  dR3mat=[0, 0; 0, 0; 0, 0]  dR4mat=[0, 0; 0, 0; 0, 0]  dR5mat=[0, 0; 0, 0; 0, 0]  prm_age_modeling=simscape.enum.tablebattery.prm_age_modeling.equation  storage_dt_age_vec=[0] d  storage_T_age_vec=[273] K  prm_age_OCV=simscape.enum.tablebattery.prm_age_OCV.OCV  OCV_age=0.9  SOC_age=0.6  prm_age_resistance=simscape.enum.tablebattery.prm_age.disabled  OCV_scaling_age_resistance=2.2134e6  OCV_offset_age_resistance=1.632e6  temp_exp_age_resistance=0.515833569 V  t_exp_age_resistance=0.75  T_age_vec_resistance=[273.15, 298.15, 323.15] K  dt_age_vec_resistance=[90, 180, 270, 360] d  dR0_age_vec=[0, 0, 0]  t_meas_dR0_age=100 d  dR0_age_mat=[0, 0, 0; 0, 0, 0; 0, 0, 0; 0, 0, 0]  prm_age_capacity=simscape.enum.tablebattery.prm_age.disabled  OCV_scaling_age_capacity=1.5097e07  OCV_offset_age_capacity=8.3625e06  temp_exp_age_capacity=0.6011 V  t_exp_age_capacity=0.75  T_age_vec_capacity=[273.15, 298.15, 323.15] K  dt_age_vec_capacity=[90, 180, 270, 360] d  dAH_age_vec=[0, 0, 0]  t_meas_dAH_age=100 d  dAH_age_mat=[0, 0, 0; 0, 0, 0; 0, 0, 0; 0, 0, 0]  thermal_port=simscape.enum.thermaleffects.model  temperature=298.15 K  thermal_mass=1 J/K  i_specify=off  i_priority=None  i=0 A  i_nominal_specify=off  i_nominal_value=1  i_nominal_unit=A  v_specify=off  v_priority=None  v=0 V  v_nominal_specify=off  v_nominal_value=1  v_nominal_unit=V  stateOfCharge_specify=on  stateOfCharge_priority=High  stateOfCharge=1  stateOfCharge_nominal_specify=on  stateOfCharge_nominal_value=1  stateOfCharge_nominal_unit=1  num_cycles_specify=off  num_cycles_priority=High  num_cycles=0  num_cycles_nominal_specify=off  num_cycles_nominal_value=1  num_cycles_nominal_unit=1  cell_temperature_specify=on  cell_temperature_priority=High  cell_temperature=298.15 K  cell_temperature_nominal_specify=off  cell_temperature_nominal_value=1  cell_temperature_nominal_unit=K
  PS-Simulink Converter2 : nesl_utility/PS-Simulink Converter  PhysicalDomain=network_engine_domain  SubClassName=ps_output  LeftPortType=input  RightPortType=output  PseudoPeriodic=off  Frequencies=[]  VectorFormat=inherit  Unit=inherit  AffineConversion=off
  PS-Simulink Converter4 : nesl_utility/PS-Simulink Converter  PhysicalDomain=network_engine_domain  SubClassName=ps_output  LeftPortType=input  RightPortType=output  PseudoPeriodic=off  Frequencies=[]  VectorFormat=inherit  Unit=inherit  AffineConversion=off
  Simulink-PS Converter{1..4} (4 alike) : nesl_utility/Simulink-PS Converter  PhysicalDomain=network_engine_domain  SubClassName=ps_input  LeftPortType=input  RightPortType=output  PseudoPeriodic=off  Frequencies=[]  NoiseDistribution=none  NoiseParameters=[]  Unit=1  AffineConversion=off  FilteringAndDerivatives=provide  SimscapeFilterOrder=1  InputFilterTimeConstant=0.001  UdotUserProvided=0
  Temperature Sensor : fl_lib/Thermal/Thermal Sensors/Temperature Sensor  temperature_measure=foundation.enum.MeasurementReference.difference
  Thermal Mass : fl_lib/Thermal/Thermal Elements/Thermal Mass  mass_type=foundation.enum.constant_variable.constant  mass=67.9 g  sp_heat=900 J/(K*kg)  mass_min=1e-6 kg  num_ports=foundation.enum.numPorts2.one  m_specify=off  m_priority=High  m=1 kg  m_nominal_specify=off  m_nominal_value=1  m_nominal_unit=kg  T_specify=off  T_priority=High  T=300 K  T_nominal_specify=off  T_nominal_value=1  T_nominal_unit=K  Q_specify=off  Q_priority=None  Q=0 W  Q_nominal_specify=off  Q_nominal_value=1  Q_nominal_unit=W
  Thermal Reference : fl_lib/Thermal/Thermal Elements/Thermal Reference
  Variable Capacitor : ee_lib/Passive/Variable Capacitor  prm=2  Cmin=1e-9 F  r=1e-6 Ohm  v0=0 V  q0=0 C
      settings: InternalSimscapePortConfiguration="{\"Bottom\":[],\"Left\":[{\"id\":\"C\",\"label\":\"C\",\"type\":\"input\"},{\"id\":\"p\",\"label\":\"+\",\"type\":\"foundation.electrical.electrical\"}],\"Right\":[{\"id\":\"n\",\"label\":\"-\",\"type\":\"foundation.electrical.electrical\"}],\"Top\":[]}"
  Variable Capacitor1 : ee_lib/Passive/Variable Capacitor  prm=2  Cmin=1e-9 F  r=1e-6 Ohm  v0=0 V  q0=0 C
      settings: InternalSimscapePortConfiguration="{\"Bottom\":[],\"Left\":[{\"id\":\"C\",\"label\":\"C\",\"type\":\"input\"},{\"id\":\"p\",\"label\":\"+\",\"type\":\"foundation.electrical.electrical\"}],\"Right\":[{\"id\":\"n\",\"label\":\"-\",\"type\":\"foundation.electrical.electrical\"}],\"Top\":[]}"
  Variable Resistor2 : fl_lib/Electrical/Electrical Elements/Variable Resistor  Rmin=0 Ohm  thermalEnable=true  thermal_mass=1 J/K  i_specify=off  i_priority=None  i=0 A  i_nominal_specify=off  i_nominal_value=1  i_nominal_unit=A  v_specify=off  v_priority=None  v=0 V  v_nominal_specify=off  v_nominal_value=1  v_nominal_unit=V  T_specify=off  T_priority=None  T=300 K  T_nominal_specify=off  T_nominal_value=1  T_nominal_unit=K
      settings: InternalSimscapePortConfiguration="{\"Bottom\":[],\"Left\":[{\"id\":\"R\",\"label\":\"R\",\"type\":\"input\"},{\"id\":\"p\",\"label\":\"+\",\"type\":\"foundation.electrical.electrical\"}],\"Right\":[{\"id\":\"n\",\"label\":\"-\",\"type\":\"foundation.electrical.electrical\"}],\"Top\":[{\"id\":\"H\",\"label\":\"H\",\"type\":\"foundation.thermal.thermal\"}]}"
  Variable Resistor3 : fl_lib/Electrical/Electrical Elements/Variable Resistor  Rmin=0 Ohm  thermalEnable=true  thermal_mass=1 J/K  i_specify=off  i_priority=None  i=0 A  i_nominal_specify=off  i_nominal_value=1  i_nominal_unit=A  v_specify=off  v_priority=None  v=0 V  v_nominal_specify=off  v_nominal_value=1  v_nominal_unit=V  T_specify=off  T_priority=None  T=300 K  T_nominal_specify=off  T_nominal_value=1  T_nominal_unit=K
      settings: InternalSimscapePortConfiguration="{\"Bottom\":[],\"Left\":[{\"id\":\"R\",\"label\":\"R\",\"type\":\"input\"},{\"id\":\"p\",\"label\":\"+\",\"type\":\"foundation.electrical.electrical\"}],\"Right\":[{\"id\":\"n\",\"label\":\"-\",\"type\":\"foundation.electrical.electrical\"}],\"Top\":[{\"id\":\"H\",\"label\":\"H\",\"type\":\"foundation.thermal.thermal\"}]}"
  Voltage Sensor : fl_lib/Electrical/Electrical Sensors/Voltage Sensor
  + : PMIOPort  Side=Right
  - : PMIOPort  Port=2  Side=Left
  V : PMIOPort  Port=3  Side=Right
  T : PMIOPort  Port=4  Side=Right
  cell_T : PMIOPort  Port=5  Side=Right
  cell_SOC : PMIOPort  Port=6  Side=Right
  wires:
  [SOC] -> 1-D Lookup Table/1
  1-D Lookup Table1/1 -> Simulink-PS Converter1/1
  PS-Simulink Converter4/1 -> [Temp]
  [Temp] -> 1-D Lookup Table3/2
  [SOC] -> 1-D Lookup Table2/1
  [SOC] -> 1-D Lookup Table1/1
  1-D Lookup Table3/1 -> Simulink-PS Converter3/1
  [SOC] -> 1-D Lookup Table3/1
  [Temp] -> 1-D Lookup Table1/2
  [Temp] -> 1-D Lookup Table2/2
  [Temp] -> 1-D Lookup Table/2
  PS-Simulink Converter2/1 -> [SOC]  "soc"
  1-D Lookup Table2/1 -> Simulink-PS Converter2/1
  1-D Lookup Table/1 -> Simulink-PS Converter4/1
  connections:
  Battery (Table-Based)/LConn2 -- cell_SOC/RConn1 -- PS-Simulink Converter2/LConn1
  Variable Capacitor/LConn2 -- Battery (Table-Based)/LConn1 -- Variable Resistor2/LConn2
  Temperature Sensor/RConn2 -- T/RConn1 -- PS-Simulink Converter4/LConn1
  -/RConn1 -- Voltage Sensor/RConn2 -- Battery (Table-Based)/RConn1
  V/RConn1 -- Voltage Sensor/RConn1
  Simulink-PS Converter3/RConn1 -- Variable Capacitor/LConn1
  Simulink-PS Converter4/RConn1 -- Variable Capacitor1/LConn1
  Thermal Reference/LConn1 -- Temperature Sensor/RConn1
  Variable Resistor3/LConn2 -- Variable Capacitor/RConn1 -- Variable Resistor2/RConn1 -- Variable Capacitor1/LConn2
  Simulink-PS Converter1/RConn1 -- Variable Resistor2/LConn1
  Simulink-PS Converter2/RConn1 -- Variable Resistor3/LConn1
  Variable Capacitor1/RConn1 -- Variable Resistor3/RConn1 -- +/RConn1 -- Voltage Sensor/LConn1
  Variable Resistor3/LConn3 -- Variable Resistor2/LConn3 -- Battery (Table-Based)/RConn2 -- Temperature Sensor/LConn1 -- cell_T/RConn1 -- Thermal Mass/LConn1
